simulink model "H8_6gdl_hil"  (R2022b)
settings: Solver=VariableStepAuto  StartTime=0.0  StopTime=10.0  RelTol=1e-3
InitFcn:
  | load("ems.mat");
  | load("hems.mat");
  | load('fuerzasY_LIM.mat')
  | load('matrices_linealizacion_6gdl.mat')
  | m = 200;
  | g = 9.81;
  | 
  | x_lev12 = 0.50086;
  | x_lev34 = 0.48414;
  | x_guid12 = 0.50503;
  | x_guid34 = 0.48831;
  | x_lim = 0.00778;
  | 
  | y_lev13 = 0.23523;
  | y_lev24 = 0.23827;
  | y_guid13 = 0.2372;
  | y_guid24 = 0.2402;
  | y_lim = 0.00154;
  | y_brk = 0.21552;
  | 
  | z_lev = 0.07138;
  | z_guid = 0.04113;
  | z_lim = 0.09146;
  | z_brk = 0.03941;
  | 
  | kp_lev = 50;
  | ki_lev = 400;
  | kp_guid = 6;
  | ki_guid = 46.5;
  | 
  | Imax_lev = 50;
  | Imin_lev = -50;
  | Imax_guid = 50;
  | Imin_guid = 0;
  | 
  | cg_nom=0.61448;
  | lev_nom=0.01965;
  | cg_suelo=0.61733;
  | cg_techo=0.60483;
  | 
  | I = [43.082 0 0; 0 26.887 -0; 0 0 29.297];
undefined symbols (not defined in the file or in its folder): current, ems, FuerzaRail_Y, hems, magnitude, Y
settings Model: Creator=aceao  LastModifiedBy=aceao

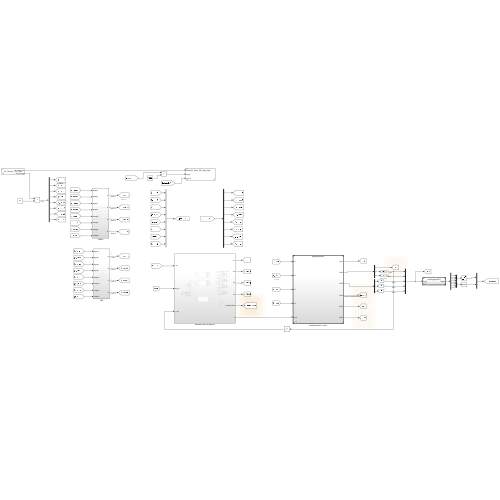
[thumbnail: Simulink's stored preview of the top-level diagram]
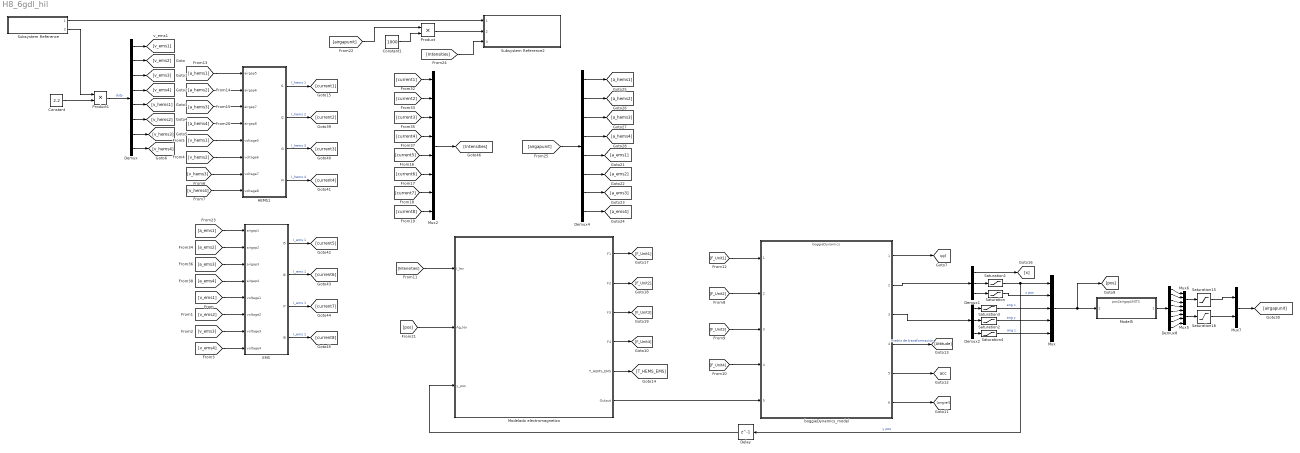
== system H8_6gdl_hil ==
  Constant : Constant  Value=2.2
  Constant1 : Constant  Value=1000
  Delay : Delay  DelayLength=1  InitialCondition=0.001
  Demux : Demux  Outputs=8
  Demux1 : Demux  Outputs=3
  Demux2 : Demux  Outputs=3
  Demux4 : Demux  Outputs=8
  Demux8 : Demux  Outputs=8
  EMS : Subsystem
  HEMS1 : Subsystem
  Model5 : ModelReference  ModelNameDialog=pos2airgapUNITS.slx  SimulationMode=Normal  ModelReferenceVersion=1.5
  Modelado electromagnetico : Subsystem
  Mux : Mux  Inputs=5
  Mux2 : Mux  Inputs=8
  Mux5 : Mux
  Mux6 : Mux
  Mux7 : Mux  Inputs=2
  Product : Product
  Product1 : Product
  Saturation : Saturate  UpperLimit=cg_suelo  LowerLimit=cg_techo
  Saturation1 : Saturate  UpperLimit=0.012  LowerLimit=-0.012
  Saturation15 : Saturate  UpperLimit=0.0225  LowerLimit=0.01
  Saturation16 : Saturate  UpperLimit=0.024  LowerLimit=0
  Saturation2 : Saturate  UpperLimit=0.01268  LowerLimit=-0.01268
  Saturation3 : Saturate  UpperLimit=0.0476  LowerLimit=-0.0476
  Saturation4 : Saturate  UpperLimit=0.024  LowerLimit=-0.024
  Subsystem Reference : Subsystem  ReferencedSubsystem=HIL_Receive_TCP_Data  mi_ip=0  mi_port=0  f=0
  Subsystem Reference2 : Subsystem  ReferencedSubsystem=HIL_Send_TCP_Data_6gdl  mi_ip=mi_ip  mi_port=mi_port  f=0
  boggieDynamics_model : ModelReference  ModelNameDialog=boggieDynamics.mdl  SimulationMode=Normal  ModelReferenceVersion=1.43
  tag scope: acc=global, vel=global
  wires:
  Mux2/1 -> [Intensities]
  [current5] -> Mux2/5
  [a_hems4] -> HEMS1/4(airgap8)
  [current2] -> Mux2/2
  HEMS1/1(I1) -> [current1]  "I_hems 1"
  [current6] -> Mux2/6
  [current7] -> Mux2/7
  [a_hems1] -> HEMS1/1(airgap5)
  HEMS1/4(I4) -> [current4]  "I_hems 4"
  [current1] -> Mux2/1
  HEMS1/2(I2) -> [current2]  "I_hems 2"
  [a_hems2] -> HEMS1/2(airgap6)
  [a_hems3] -> HEMS1/3(airgap7)
  [current3] -> Mux2/3
  HEMS1/3(I3) -> [current3]  "I_hems 3"
  [current8] -> Mux2/8
  [current4] -> Mux2/4
  Subsystem Reference/1 -> Subsystem Reference2/1
  [a_ems3] -> EMS/3(airgap3)
  [a_ems1] -> EMS/1(airgap1)
  [a_ems4] -> EMS/4(airgap4)
  [a_ems2] -> EMS/2(airgap2)
  EMS/4(I8) -> [current8]  "I_ems 1"
  EMS/3(I7) -> [current7]  "I_ems 1"
  EMS/1(I5) -> [current5]  "I_ems 1"
  EMS/2(I6) -> [current6]  "I_ems 1"
  Product1/1 -> Demux/1  "duty"
  Subsystem Reference/2 -> Product1/1
  Constant/1 -> Product1/2
  [v_ems1] -> EMS/5(voltage1)
  [v_ems2] -> EMS/6(voltage2)
  [v_ems3] -> EMS/7(voltage3)
  [v_ems4] -> EMS/8(voltage4)
  Demux/1 -> [v_ems1]
  Demux/2 -> [v_ems2]
  Demux/3 -> [v_ems3]
  Demux/4 -> [v_ems4]
  Demux/5 -> [v_hems1]
  Demux/6 -> [v_hems2]
  [v_hems1] -> HEMS1/5(voltage5)
  [v_hems2] -> HEMS1/6(voltage6)
  [v_hems3] -> HEMS1/7(voltage7)
  Demux/7 -> [v_hems3]
  [v_hems4] -> HEMS1/8(voltage8)
  Demux/8 -> [v_hems4]
  Modelado electromagnetico/3(F3) -> [F_Unit3]
  boggieDynamics_model/6 -> [angvel]
  Demux1/2 -> Saturation1/1
  Delay/1 -> Modelado electromagnetico/3(y_pos)
  Modelado electromagnetico/6(Output) -> boggieDynamics_model/5
  Demux2/1 -> Saturation3/1
  Saturation2/1 -> Mux/4  "ang y"
  [Intensities] -> Modelado electromagnetico/1(I_lev)
  Saturation4/1 -> Mux/5  "ang z"
  Saturation1/1 -> Delay/1, Mux/1  "y pos"
  boggieDynamics_model/2 -> Demux1/1
  Demux2/2 -> Saturation2/1
  Modelado electromagnetico/1(F1) -> [F_Unit1]
  Saturation3/1 -> Mux/3  "ang x"
  Modelado electromagnetico/5(T_HEMS_EMS) -> [T_HEMS_EMS]
  boggieDynamics_model/5 -> [acc]
  [F_Unit2] -> boggieDynamics_model/2
  Saturation/1 -> Mux/2  "z pos"
  Mux/1 -> Model5/1, [pos]
  boggieDynamics_model/4 -> [Attitude]  "matriz de transformacion"
  [F_Unit1] -> boggieDynamics_model/1
  Demux1/3 -> Saturation/1
  [F_Unit3] -> boggieDynamics_model/3
  Demux2/3 -> Saturation4/1
  [pos] -> Modelado electromagnetico/2(Ag_lev)
  Modelado electromagnetico/4(F4) -> [F_Unit4]
  Modelado electromagnetico/2(F2) -> [F_Unit2]
  [F_Unit4] -> boggieDynamics_model/4
  Demux1/1 -> [x]
  boggieDynamics_model/3 -> Demux2/1
  boggieDynamics_model/1 -> [vel]
  [Intensities] -> Subsystem Reference2/3
  Demux4/8 -> [a_ems4]
  Demux4/4 -> [a_hems4]
  Demux4/5 -> [a_ems1]
  [airgapunit] -> Demux4/1
  Demux4/6 -> [a_ems2]
  Demux4/3 -> [a_hems3]
  Demux4/2 -> [a_hems2]
  Demux4/1 -> [a_hems1]
  Demux4/7 -> [a_ems3]
  Mux7/1 -> [airgapunit]
  Demux8/6 -> Mux5/2
  Demux8/8 -> Mux5/4
  Demux8/1 -> Mux6/1
  Demux8/4 -> Mux6/4
  Model5/1 -> Demux8/1
  Demux8/7 -> Mux5/3
  Saturation15/1 -> Mux7/1
  Demux8/3 -> Mux6/3
  Mux5/1 -> Saturation16/1
  Mux6/1 -> Saturation15/1
  Demux8/5 -> Mux5/1
  Demux8/2 -> Mux6/2
  Saturation16/1 -> Mux7/2
  Constant1/1 -> Product/2
  [airgapunit] -> Product/1
  Product/1 -> Subsystem Reference2/2

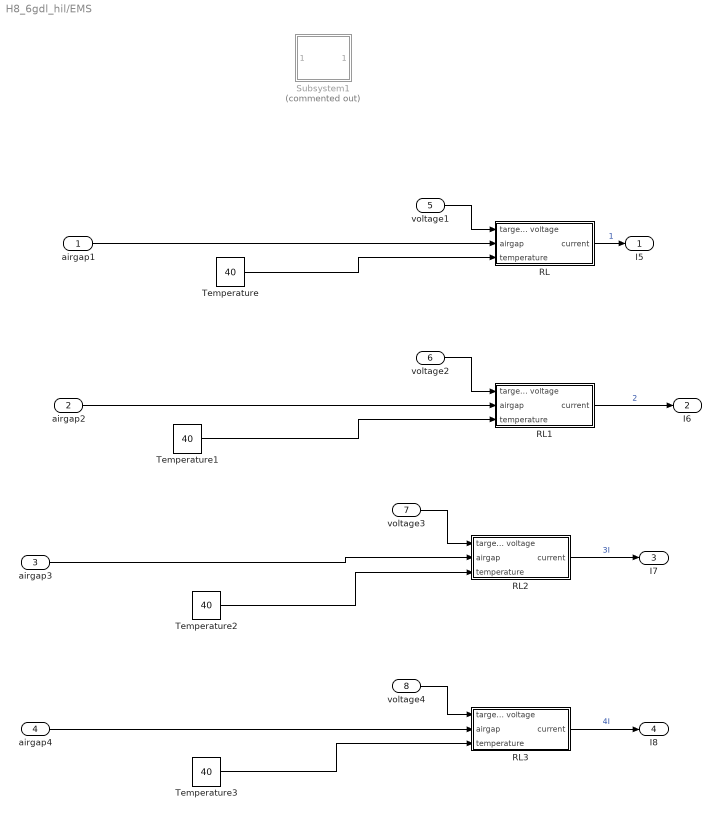
== system H8_6gdl_hil/EMS ==
  airgap1 : Inport
  airgap2 : Inport  Port=2
  airgap3 : Inport  Port=3
  airgap4 : Inport  Port=4
  voltage1 : Inport  Port=5
  voltage2 : Inport  Port=6
  voltage3 : Inport  Port=7
  voltage4 : Inport  Port=8
  RL : Subsystem
  RL1 : Subsystem
  RL2 : Subsystem
  RL3 : Subsystem
  Subsystem1 : Subsystem  Commented=on
  Temperature{,1..3} (4 alike) : Constant  Value=40
  I5 : Outport
  I6 : Outport  Port=2
  I7 : Outport  Port=3
  I8 : Outport  Port=4
  wires:
  Temperature/1 -> RL/3(temperature)
  airgap1/1 -> RL/2(airgap)
  Temperature3/1 -> RL3/3(temperature)
  RL/1(current) -> I5/1  "1"
  Temperature1/1 -> RL1/3(temperature)
  Temperature2/1 -> RL2/3(temperature)
  RL3/1(current) -> I8/1  "4I"
  airgap2/1 -> RL1/2(airgap)
  RL1/1(current) -> I6/1  "2"
  RL2/1(current) -> I7/1  "3I"
  airgap3/1 -> RL2/2(airgap)
  airgap4/1 -> RL3/2(airgap)
  voltage2/1 -> RL1/1(target voltage)
  voltage3/1 -> RL2/1(target voltage)
  voltage1/1 -> RL/1(target voltage)
  voltage4/1 -> RL3/1(target voltage)

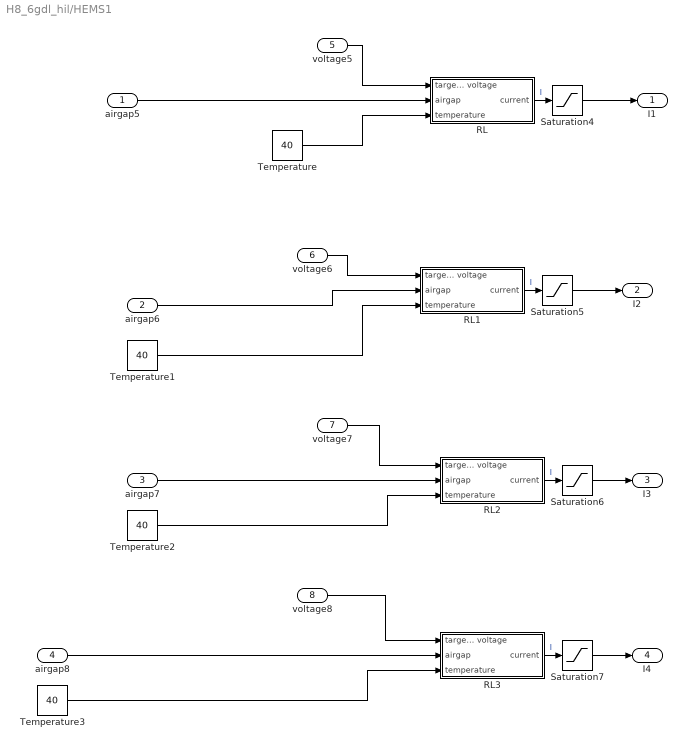
== system H8_6gdl_hil/HEMS1 ==
  airgap5 : Inport
  airgap6 : Inport  Port=2
  airgap7 : Inport  Port=3
  airgap8 : Inport  Port=4
  voltage5 : Inport  Port=5
  voltage6 : Inport  Port=6
  voltage7 : Inport  Port=7
  voltage8 : Inport  Port=8
  RL : Subsystem
  RL1 : Subsystem
  RL2 : Subsystem
  RL3 : Subsystem
  Saturation{4..7} (4 alike) : Saturate  UpperLimit=50  LowerLimit=-50
  Temperature{,1..3} (4 alike) : Constant  Value=40
  I1 : Outport
  I2 : Outport  Port=2
  I3 : Outport  Port=3
  I4 : Outport  Port=4
  wires:
  Temperature/1 -> RL/3(temperature)
  airgap5/1 -> RL/2(airgap)
  Temperature3/1 -> RL3/3(temperature)
  RL/1(current) -> Saturation4/1  "I"
  Temperature1/1 -> RL1/3(temperature)
  Temperature2/1 -> RL2/3(temperature)
  RL3/1(current) -> Saturation7/1  "I"
  airgap6/1 -> RL1/2(airgap)
  RL1/1(current) -> Saturation5/1  "I"
  RL2/1(current) -> Saturation6/1  "I"
  airgap7/1 -> RL2/2(airgap)
  airgap8/1 -> RL3/2(airgap)
  Saturation4/1 -> I1/1
  Saturation5/1 -> I2/1
  Saturation7/1 -> I4/1
  Saturation6/1 -> I3/1
  voltage5/1 -> RL/1(target voltage)
  voltage6/1 -> RL1/1(target voltage)
  voltage7/1 -> RL2/1(target voltage)
  voltage8/1 -> RL3/1(target voltage)

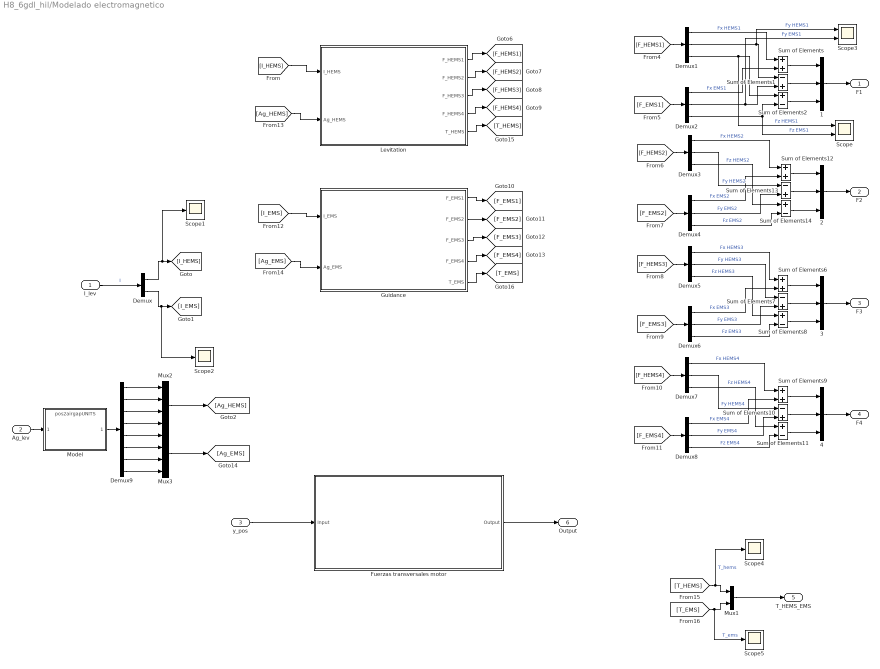
== system H8_6gdl_hil/Modelado electromagnetico ==
  I_lev : Inport
  Ag_lev : Inport  Port=2
  y_pos : Inport  Port=3
  {1..4} (4 alike) : Mux  Inputs=3
  Demux : Demux  Outputs=2
  Demux{1..8} (8 alike) : Demux  Outputs=3
  Demux9 : Demux  Outputs=8
  Fuerzas transversales motor : Subsystem
  Guidance : Subsystem
  Levitation : Subsystem
  Model : ModelReference  ModelNameDialog=pos2airgapUNITS.slx  SimulationMode=Normal  ModelReferenceVersion=1.5
  Mux1 : Mux  Inputs=2
  Mux2 : Mux
  Mux3 : Mux
  Scope : Scope  NumInputPorts=2
  Scope{1..2,4..5} (4 alike) : Scope
  Scope3 : Scope  NumInputPorts=2
  Sum of Elements{,6,9,12} (4 alike) : Sum
  Sum of Elements{1,7,10,13} (4 alike) : Sum  Inputs=-+
  Sum of Elements{2,8,11,14} (4 alike) : Sum  Inputs=+-
  F1 : Outport
  F2 : Outport  Port=2
  F3 : Outport  Port=3
  F4 : Outport  Port=4
  T_HEMS_EMS : Outport  Port=5
  Output : Outport  Port=6
  wires:
  I_lev/1 -> Demux/1  "I"
  Demux/1 -> Scope1/1, [I_HEMS]
  Demux/2 -> Scope2/1, [I_EMS]
  [I_HEMS] -> Levitation/1(I_HEMS)
  Levitation/1(F_HEMS1) -> [F_HEMS1]
  Levitation/2(F_HEMS2) -> [F_HEMS2]
  Levitation/3(F_HEMS3) -> [F_HEMS3]
  Levitation/4(F_HEMS4) -> [F_HEMS4]
  Sum of Elements/1 -> 1/1
  1/1 -> F1/1
  Sum of Elements1/1 -> 1/2
  Sum of Elements2/1 -> 1/3
  2/1 -> F2/1
  [F_HEMS1] -> Demux1/1
  Demux1/1 -> Sum of Elements/1  "Fx HEMS1"
  Demux1/2 -> Scope3/1, Sum of Elements1/1  "Fy HEMS1"
  Demux1/3 -> Scope/1, Sum of Elements2/1  "Fz HEMS1"
  3/1 -> F3/1
  Sum of Elements8/1 -> 3/3
  Sum of Elements6/1 -> 3/1
  Sum of Elements7/1 -> 3/2
  4/1 -> F4/1
  Sum of Elements11/1 -> 4/3
  Sum of Elements9/1 -> 4/1
  Sum of Elements10/1 -> 4/2
  Guidance/2(F_EMS2) -> [F_EMS2]
  Guidance/3(F_EMS3) -> [F_EMS3]
  Guidance/4(F_EMS4) -> [F_EMS4]
  Guidance/1(F_EMS1) -> [F_EMS1]
  Demux2/1 -> Sum of Elements/2  "Fx EMS1"
  [F_EMS1] -> Demux2/1
  Demux2/2 -> Scope3/2, Sum of Elements1/2  "Fy EMS1"
  Demux2/3 -> Sum of Elements2/2, Scope/2  "Fz EMS1"
  [F_EMS2] -> Demux4/1
  Demux4/1 -> Sum of Elements12/2  "Fx EMS2"
  Demux4/2 -> Sum of Elements13/2  "Fy EMS2"
  Sum of Elements14/1 -> 2/3
  Demux3/1 -> Sum of Elements12/1  "Fx HEMS2"
  [F_HEMS2] -> Demux3/1
  Demux3/2 -> Sum of Elements13/1  "Fy HEMS2"
  Demux3/3 -> Sum of Elements14/1  "Fz HEMS2"
  Sum of Elements13/1 -> 2/2
  Sum of Elements12/1 -> 2/1
  Demux4/3 -> Sum of Elements14/2  "Fz EMS2"
  Demux5/3 -> Sum of Elements8/1  "Fz HEMS3"
  Demux5/2 -> Sum of Elements7/1  "Fy HEMS3"
  [F_HEMS3] -> Demux5/1
  Demux6/3 -> Sum of Elements8/2  "Fz EMS3"
  [F_EMS3] -> Demux6/1
  Demux6/1 -> Sum of Elements6/2  "Fx EMS3"
  Demux5/1 -> Sum of Elements6/1  "Fx HEMS3"
  Demux6/2 -> Sum of Elements7/2  "Fy EMS3"
  Demux7/3 -> Sum of Elements11/1  "Fz HEMS4"
  Demux8/3 -> Sum of Elements11/2  "Fz EMS4"
  Demux8/2 -> Sum of Elements10/2  "Fy EMS4"
  Demux7/2 -> Sum of Elements10/1  "Fy HEMS4"
  Demux7/1 -> Sum of Elements9/1  "Fx HEMS4"
  Demux8/1 -> Sum of Elements9/2  "Fx EMS4"
  [F_HEMS4] -> Demux7/1
  [F_EMS4] -> Demux8/1
  [I_EMS] -> Guidance/1(I_EMS)
  Ag_lev/1 -> Model/1
  [Ag_HEMS] -> Levitation/2(Ag_HEMS)
  [Ag_EMS] -> Guidance/2(Ag_EMS)
  Levitation/5(T_HEMS) -> [T_HEMS]
  Guidance/5(T_EMS) -> [T_EMS]
  Mux1/1 -> T_HEMS_EMS/1
  [T_HEMS] -> Scope4/1, Mux1/1  "T_hems"
  [T_EMS] -> Scope5/1, Mux1/2  "T_ems"
  Model/1 -> Demux9/1
  Demux9/1 -> Mux2/1
  Demux9/2 -> Mux2/2
  Demux9/3 -> Mux2/3
  Demux9/4 -> Mux2/4
  Mux2/1 -> [Ag_HEMS]
  Demux9/5 -> Mux3/1
  Demux9/7 -> Mux3/3
  Mux3/1 -> [Ag_EMS]
  Demux9/6 -> Mux3/2
  Demux9/8 -> Mux3/4
  y_pos/1 -> Fuerzas transversales motor/1(Input)
  Fuerzas transversales motor/1(Output) -> Output/1

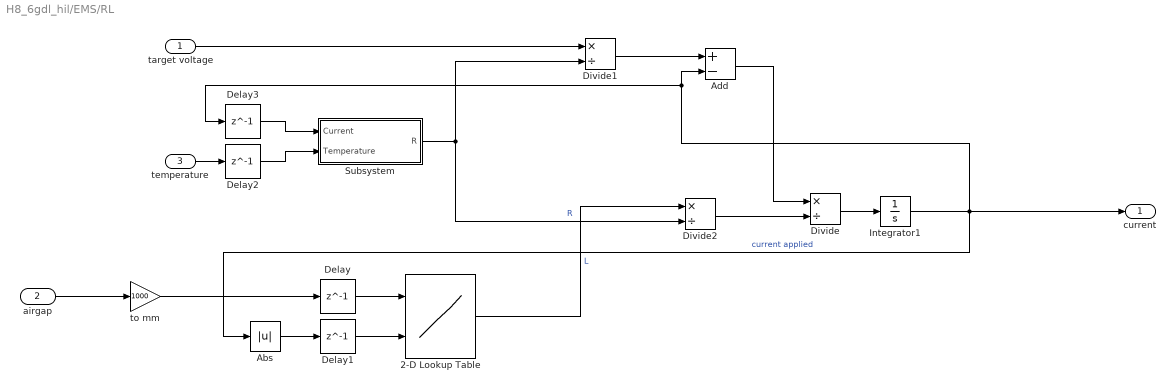
== system H8_6gdl_hil/EMS/RL ==
  target voltage : Inport
  airgap : Inport  Port=2
  temperature : Inport  Port=3
  2-D Lookup Table : Lookup_n-D  BreakpointsForDimension1=ems.Airgap  BreakpointsForDimension2=ems.Flux_Current(2:55)  Table=ems.Inductance  InternalRulePriority=Speed  RndMeth=Simplest
      settings: InputPortMap=u0,u1
  Abs : Abs  SaturateOnIntegerOverflow=off
  Add : Sum  Inputs=+-
  Delay{,1..3} (4 alike) : Delay  DelayLength=1
  Divide : Product  Inputs=*/
  Divide1 : Product  Inputs=*/
  Divide2 : Product  Inputs=*/
  Integrator1 : Integrator
  Subsystem : Subsystem
  to mm : Gain  Gain=1000
  current : Outport
  wires:
  airgap/1 -> to mm/1
  Divide/1 -> Integrator1/1
  Add/1 -> Divide/1
  Integrator1/1 -> Abs/1, current/1, Delay3/1, Add/2  "current applied"
  2-D Lookup Table/1 -> Divide2/1  "L"
  target voltage/1 -> Divide1/1
  temperature/1 -> Delay2/1
  Divide1/1 -> Add/1
  Subsystem/1(R) -> Divide2/2, Divide1/2  "R"
  Delay3/1 -> Subsystem/1(Current)
  Delay2/1 -> Subsystem/2(Temperature)
  Divide2/1 -> Divide/2
  Delay1/1 -> 2-D Lookup Table/2
  Delay/1 -> 2-D Lookup Table/1
  Abs/1 -> Delay1/1
  to mm/1 -> Delay/1

== system H8_6gdl_hil/EMS/RL1 ==
  target voltage : Inport
  airgap : Inport  Port=2
  temperature : Inport  Port=3
  2-D Lookup Table : Lookup_n-D  BreakpointsForDimension1=ems.Airgap  BreakpointsForDimension2=ems.Flux_Current(2:55)  Table=ems.Inductance  InternalRulePriority=Speed  RndMeth=Simplest
      settings: InputPortMap=u0,u1
  Abs : Abs  SaturateOnIntegerOverflow=off
  Add : Sum  Inputs=+-
  Delay{,1..3} (4 alike) : Delay  DelayLength=1
  Divide : Product  Inputs=*/
  Divide1 : Product  Inputs=*/
  Divide2 : Product  Inputs=*/
  Integrator1 : Integrator
  Subsystem : Subsystem
  to mm : Gain  Gain=1000
  current : Outport
  wires:
  airgap/1 -> to mm/1
  Divide/1 -> Integrator1/1
  Add/1 -> Divide/1
  Integrator1/1 -> Abs/1, current/1, Delay3/1, Add/2  "current applied"
  2-D Lookup Table/1 -> Divide2/1  "L"
  target voltage/1 -> Divide1/1
  temperature/1 -> Delay2/1
  Divide1/1 -> Add/1
  Subsystem/1(R) -> Divide2/2, Divide1/2  "R"
  Delay3/1 -> Subsystem/1(Current)
  Delay2/1 -> Subsystem/2(Temperature)
  Divide2/1 -> Divide/2
  Delay1/1 -> 2-D Lookup Table/2
  Delay/1 -> 2-D Lookup Table/1
  Abs/1 -> Delay1/1
  to mm/1 -> Delay/1

== system H8_6gdl_hil/EMS/RL2 ==
  target voltage : Inport
  airgap : Inport  Port=2
  temperature : Inport  Port=3
  2-D Lookup Table : Lookup_n-D  BreakpointsForDimension1=ems.Airgap  BreakpointsForDimension2=ems.Flux_Current(2:55)  Table=ems.Inductance  InternalRulePriority=Speed  RndMeth=Simplest
      settings: InputPortMap=u0,u1
  Abs : Abs  SaturateOnIntegerOverflow=off
  Add : Sum  Inputs=+-
  Delay{,1..3} (4 alike) : Delay  DelayLength=1
  Divide : Product  Inputs=*/
  Divide1 : Product  Inputs=*/
  Divide2 : Product  Inputs=*/
  Integrator1 : Integrator
  Subsystem : Subsystem
  to mm : Gain  Gain=1000
  current : Outport
  wires:
  airgap/1 -> to mm/1
  Divide/1 -> Integrator1/1
  Add/1 -> Divide/1
  Integrator1/1 -> Abs/1, current/1, Delay3/1, Add/2  "current applied"
  2-D Lookup Table/1 -> Divide2/1  "L"
  target voltage/1 -> Divide1/1
  temperature/1 -> Delay2/1
  Divide1/1 -> Add/1
  Subsystem/1(R) -> Divide2/2, Divide1/2  "R"
  Delay3/1 -> Subsystem/1(Current)
  Delay2/1 -> Subsystem/2(Temperature)
  Divide2/1 -> Divide/2
  Delay1/1 -> 2-D Lookup Table/2
  Delay/1 -> 2-D Lookup Table/1
  Abs/1 -> Delay1/1
  to mm/1 -> Delay/1

== system H8_6gdl_hil/EMS/RL3 ==
  target voltage : Inport
  airgap : Inport  Port=2
  temperature : Inport  Port=3
  2-D Lookup Table : Lookup_n-D  BreakpointsForDimension1=ems.Airgap  BreakpointsForDimension2=ems.Flux_Current(2:55)  Table=ems.Inductance  InternalRulePriority=Speed  RndMeth=Simplest
      settings: InputPortMap=u0,u1
  Abs : Abs  SaturateOnIntegerOverflow=off
  Add : Sum  Inputs=+-
  Delay{,1..3} (4 alike) : Delay  DelayLength=1
  Divide : Product  Inputs=*/
  Divide1 : Product  Inputs=*/
  Divide2 : Product  Inputs=*/
  Integrator1 : Integrator
  Subsystem : Subsystem
  to mm : Gain  Gain=1000
  current : Outport
  wires:
  airgap/1 -> to mm/1
  Divide/1 -> Integrator1/1
  Add/1 -> Divide/1
  Integrator1/1 -> Abs/1, current/1, Delay3/1, Add/2  "current applied"
  2-D Lookup Table/1 -> Divide2/1  "L"
  target voltage/1 -> Divide1/1
  temperature/1 -> Delay2/1
  Divide1/1 -> Add/1
  Subsystem/1(R) -> Divide2/2, Divide1/2  "R"
  Delay3/1 -> Subsystem/1(Current)
  Delay2/1 -> Subsystem/2(Temperature)
  Divide2/1 -> Divide/2
  Delay1/1 -> 2-D Lookup Table/2
  Delay/1 -> 2-D Lookup Table/1
  Abs/1 -> Delay1/1
  to mm/1 -> Delay/1

== system H8_6gdl_hil/EMS/Subsystem1 ==
  current5 : Inport
  Constant : Constant  Value=0
  Constant2 : Constant  Value=50
  Switch : Switch  Criteria=u2 > Threshold  SaturateOnIntegerOverflow=off  InputSameDT=off
  Switch1 : Switch  Criteria=u2 > Threshold  Threshold=50  SaturateOnIntegerOverflow=off  InputSameDT=off
  Out1 : Outport
  wires:
  current5/1 -> Switch/1, Switch/2
  Switch1/1 -> Out1/1
  Switch/1 -> Switch1/3, Switch1/2
  Constant/1 -> Switch/3
  Constant2/1 -> Switch1/1

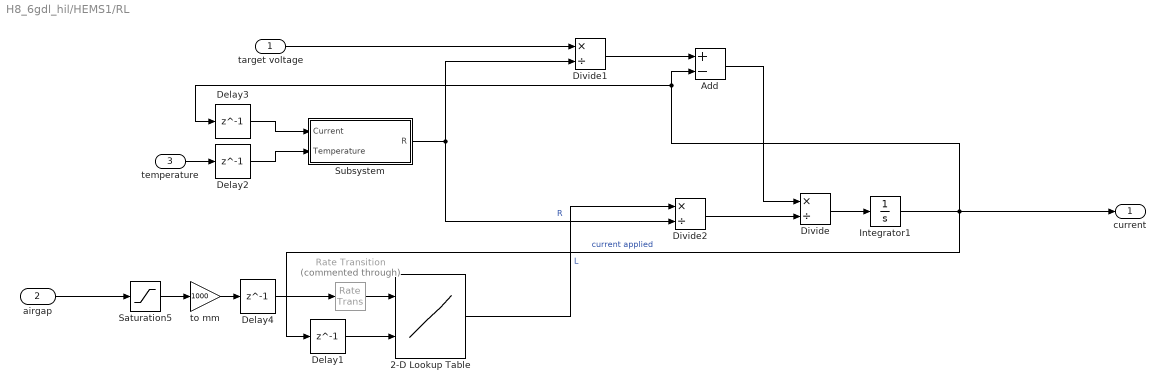
== system H8_6gdl_hil/HEMS1/RL ==
  target voltage : Inport
  airgap : Inport  Port=2
  temperature : Inport  Port=3
  2-D Lookup Table : Lookup_n-D  BreakpointsForDimension1=hems.Airgap  BreakpointsForDimension2=hems.Current(2:110)  Table=hems.Inductance  InternalRulePriority=Speed  RndMeth=Simplest
      settings: InputPortMap=u0,u1
  Add : Sum  Inputs=+-
  Delay{1..4} (4 alike) : Delay  DelayLength=1
  Divide : Product  Inputs=*/
  Divide1 : Product  Inputs=*/
  Divide2 : Product  Inputs=*/
  Integrator1 : Integrator
  Rate Transition : RateTransition  Commented=through
  Saturation5 : Saturate  UpperLimit=0.0225  LowerLimit=0.01
  Subsystem : Subsystem
  to mm : Gain  Gain=1000
  current : Outport
  wires:
  airgap/1 -> Saturation5/1
  Divide/1 -> Integrator1/1
  Add/1 -> Divide/1
  Integrator1/1 -> Delay1/1, current/1, Delay3/1, Add/2  "current applied"
  2-D Lookup Table/1 -> Divide2/1  "L"
  temperature/1 -> Delay2/1
  Divide1/1 -> Add/1
  Subsystem/1(R) -> Divide2/2, Divide1/2  "R"
  Delay3/1 -> Subsystem/1(Current)
  Delay2/1 -> Subsystem/2(Temperature)
  Divide2/1 -> Divide/2
  Delay1/1 -> 2-D Lookup Table/2
  Rate Transition/1 -> 2-D Lookup Table/1
  Saturation5/1 -> to mm/1
  to mm/1 -> Delay4/1
  Delay4/1 -> Rate Transition/1
  target voltage/1 -> Divide1/1

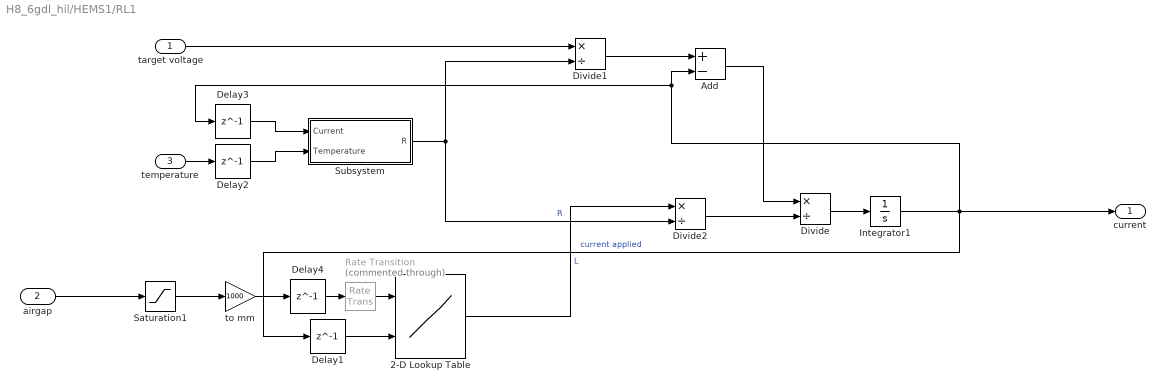
== system H8_6gdl_hil/HEMS1/RL1 ==
  target voltage : Inport
  airgap : Inport  Port=2
  temperature : Inport  Port=3
  2-D Lookup Table : Lookup_n-D  BreakpointsForDimension1=hems.Airgap  BreakpointsForDimension2=hems.Current(2:110)  Table=hems.Inductance  InternalRulePriority=Speed  RndMeth=Simplest
      settings: InputPortMap=u0,u1
  Add : Sum  Inputs=+-
  Delay{1..4} (4 alike) : Delay  DelayLength=1
  Divide : Product  Inputs=*/
  Divide1 : Product  Inputs=*/
  Divide2 : Product  Inputs=*/
  Integrator1 : Integrator
  Rate Transition : RateTransition  Commented=through
  Saturation1 : Saturate  UpperLimit=0.0225  LowerLimit=0.01
  Subsystem : Subsystem
  to mm : Gain  Gain=1000
  current : Outport
  wires:
  airgap/1 -> Saturation1/1
  Divide/1 -> Integrator1/1
  Add/1 -> Divide/1
  Integrator1/1 -> Delay1/1, current/1, Delay3/1, Add/2  "current applied"
  2-D Lookup Table/1 -> Divide2/1  "L"
  target voltage/1 -> Divide1/1
  temperature/1 -> Delay2/1
  Divide1/1 -> Add/1
  Subsystem/1(R) -> Divide2/2, Divide1/2  "R"
  Delay3/1 -> Subsystem/1(Current)
  Delay2/1 -> Subsystem/2(Temperature)
  Divide2/1 -> Divide/2
  Delay1/1 -> 2-D Lookup Table/2
  Rate Transition/1 -> 2-D Lookup Table/1
  Saturation1/1 -> to mm/1
  to mm/1 -> Delay4/1
  Delay4/1 -> Rate Transition/1

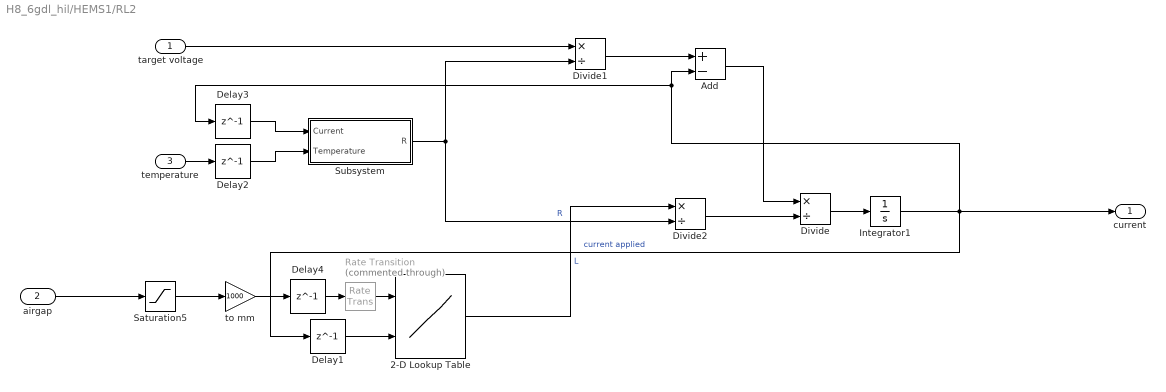
== system H8_6gdl_hil/HEMS1/RL2 ==
  target voltage : Inport
  airgap : Inport  Port=2
  temperature : Inport  Port=3
  2-D Lookup Table : Lookup_n-D  BreakpointsForDimension1=hems.Airgap  BreakpointsForDimension2=hems.Current(2:110)  Table=hems.Inductance  InternalRulePriority=Speed  RndMeth=Simplest
      settings: InputPortMap=u0,u1
  Add : Sum  Inputs=+-
  Delay{1..4} (4 alike) : Delay  DelayLength=1
  Divide : Product  Inputs=*/
  Divide1 : Product  Inputs=*/
  Divide2 : Product  Inputs=*/
  Integrator1 : Integrator
  Rate Transition : RateTransition  Commented=through
  Saturation5 : Saturate  UpperLimit=0.0225  LowerLimit=0.01
  Subsystem : Subsystem
  to mm : Gain  Gain=1000
  current : Outport
  wires:
  airgap/1 -> Saturation5/1
  Divide/1 -> Integrator1/1
  Add/1 -> Divide/1
  Integrator1/1 -> Delay1/1, current/1, Delay3/1, Add/2  "current applied"
  2-D Lookup Table/1 -> Divide2/1  "L"
  target voltage/1 -> Divide1/1
  temperature/1 -> Delay2/1
  Divide1/1 -> Add/1
  Subsystem/1(R) -> Divide2/2, Divide1/2  "R"
  Delay3/1 -> Subsystem/1(Current)
  Delay2/1 -> Subsystem/2(Temperature)
  Divide2/1 -> Divide/2
  Delay1/1 -> 2-D Lookup Table/2
  Rate Transition/1 -> 2-D Lookup Table/1
  Saturation5/1 -> to mm/1
  to mm/1 -> Delay4/1
  Delay4/1 -> Rate Transition/1

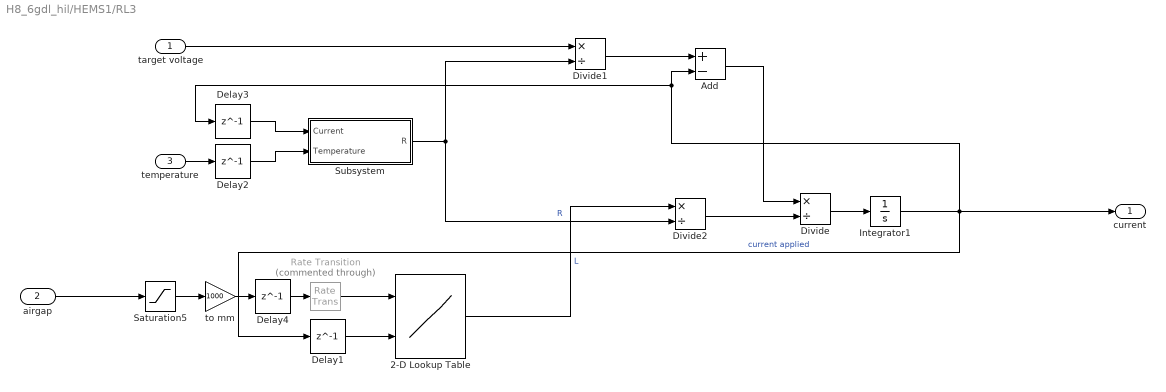
== system H8_6gdl_hil/HEMS1/RL3 ==
  target voltage : Inport
  airgap : Inport  Port=2
  temperature : Inport  Port=3
  2-D Lookup Table : Lookup_n-D  BreakpointsForDimension1=hems.Airgap  BreakpointsForDimension2=hems.Current(2:110)  Table=hems.Inductance  InternalRulePriority=Speed  RndMeth=Simplest
      settings: InputPortMap=u0,u1
  Add : Sum  Inputs=+-
  Delay{1..4} (4 alike) : Delay  DelayLength=1
  Divide : Product  Inputs=*/
  Divide1 : Product  Inputs=*/
  Divide2 : Product  Inputs=*/
  Integrator1 : Integrator
  Rate Transition : RateTransition  Commented=through
  Saturation5 : Saturate  UpperLimit=0.0225  LowerLimit=0.01
  Subsystem : Subsystem
  to mm : Gain  Gain=1000
  current : Outport
  wires:
  airgap/1 -> Saturation5/1
  Divide/1 -> Integrator1/1
  Add/1 -> Divide/1
  Integrator1/1 -> Delay1/1, current/1, Delay3/1, Add/2  "current applied"
  2-D Lookup Table/1 -> Divide2/1  "L"
  target voltage/1 -> Divide1/1
  temperature/1 -> Delay2/1
  Divide1/1 -> Add/1
  Subsystem/1(R) -> Divide2/2, Divide1/2  "R"
  Delay3/1 -> Subsystem/1(Current)
  Delay2/1 -> Subsystem/2(Temperature)
  Divide2/1 -> Divide/2
  Delay1/1 -> 2-D Lookup Table/2
  Rate Transition/1 -> 2-D Lookup Table/1
  Saturation5/1 -> to mm/1
  to mm/1 -> Delay4/1
  Delay4/1 -> Rate Transition/1

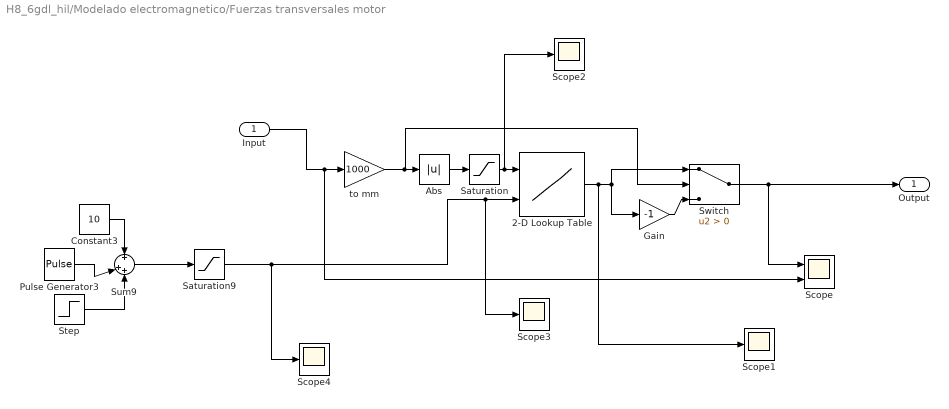
== system H8_6gdl_hil/Modelado electromagnetico/Fuerzas transversales motor ==
  Input : Inport
  2-D Lookup Table : Lookup_n-D  BreakpointsForDimension1=Y  BreakpointsForDimension2=current  Table=FuerzaRail_Y  InternalRulePriority=Speed  RndMeth=Simplest
      settings: InputPortMap=u0,u1
  Abs : Abs  SaturateOnIntegerOverflow=off
  Constant3 : Constant  Value=10
  Gain : Gain  Gain=-1
  Pulse Generator3 : DiscretePulseGenerator  PulseType=Time based  Amplitude=100  PulseWidth=95  PhaseDelay=1
  Saturation : Saturate  UpperLimit=6  LowerLimit=0
  Saturation9 : Saturate  UpperLimit=100  LowerLimit=0
  Scope : Scope  NumInputPorts=2
  Scope{1..4} (4 alike) : Scope
  Step : Step  Time=5  After=-100  SampleTime=0
  Sum9 : Sum  Inputs=+|++
  Switch : Switch  Criteria=u2 > Threshold  SaturateOnIntegerOverflow=off  InputSameDT=off
  to mm : Gain  Gain=1000
  Output : Outport
  wires:
  Input/1 -> to mm/1, Scope/2
  Gain/1 -> Switch/3
  Abs/1 -> Saturation/1
  to mm/1 -> Switch/2, Abs/1
  2-D Lookup Table/1 -> Scope1/1, Gain/1, Switch/1
  Saturation9/1 -> Scope4/1, Scope3/1, 2-D Lookup Table/2
  Switch/1 -> Output/1, Scope/1
  Saturation/1 -> Scope2/1, 2-D Lookup Table/1
  Sum9/1 -> Saturation9/1
  Pulse Generator3/1 -> Sum9/2
  Constant3/1 -> Sum9/1
  Step/1 -> Sum9/3

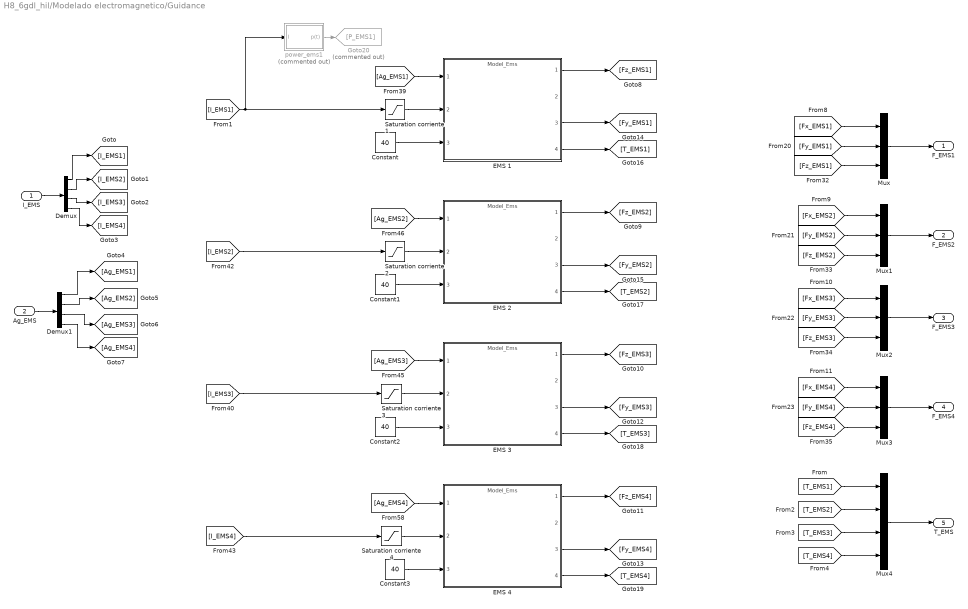
== system H8_6gdl_hil/Modelado electromagnetico/Guidance ==
  I_EMS : Inport
  Ag_EMS : Inport  Port=2
  Constant{,1..3} (4 alike) : Constant  Value=40
  Demux : Demux
  Demux1 : Demux
  EMS {1..4} (4 alike) : ModelReference  ModelNameDialog=Model_Ems.slx  SimulationMode=Normal  ModelReferenceVersion=1.23
  Goto20 : Goto  Commented=on  GotoTag=P_EMS1
  Mux{,1..3} (4 alike) : Mux  Inputs=3
  Mux4 : Mux
  Saturation corriente {1..4} (4 alike) : Saturate  UpperLimit=Imax_guid  LowerLimit=Imin_guid
  power_ems1 : Subsystem  Commented=on
  F_EMS1 : Outport
  F_EMS2 : Outport  Port=2
  F_EMS3 : Outport  Port=3
  F_EMS4 : Outport  Port=4
  T_EMS : Outport  Port=5
  wires:
  [Fz_EMS4] -> Mux3/3
  Demux1/4 -> [Ag_EMS4]
  [Fy_EMS1] -> Mux/2
  I_EMS/1 -> Demux/1
  Mux1/1 -> F_EMS2/1
  Demux/2 -> [I_EMS2]
  [Fy_EMS3] -> Mux2/2
  Mux3/1 -> F_EMS4/1
  [Fy_EMS4] -> Mux3/2
  [Fz_EMS1] -> Mux/3
  Mux/1 -> F_EMS1/1
  Mux2/1 -> F_EMS3/1
  [Fx_EMS3] -> Mux2/1
  Demux1/3 -> [Ag_EMS3]
  Ag_EMS/1 -> Demux1/1
  [Fz_EMS3] -> Mux2/3
  Demux/1 -> [I_EMS1]
  [Fz_EMS2] -> Mux1/3
  [Fx_EMS1] -> Mux/1
  Demux1/1 -> [Ag_EMS1]
  Demux/4 -> [I_EMS4]
  [Fx_EMS2] -> Mux1/1
  [Fy_EMS2] -> Mux1/2
  [Fx_EMS4] -> Mux3/1
  Demux/3 -> [I_EMS3]
  Demux1/2 -> [Ag_EMS2]
  EMS 1/3 -> [Fy_EMS1]
  [Ag_EMS4] -> EMS 4/1
  EMS 4/3 -> [Fy_EMS4]
  EMS 4/1 -> [Fz_EMS4]
  EMS 2/1 -> [Fz_EMS2]
  EMS 3/1 -> [Fz_EMS3]
  [Ag_EMS3] -> EMS 3/1
  Constant1/1 -> EMS 2/3
  Constant3/1 -> EMS 4/3
  Constant2/1 -> EMS 3/3
  Constant/1 -> EMS 1/3
  EMS 1/1 -> [Fz_EMS1]
  [Ag_EMS2] -> EMS 2/1
  EMS 3/3 -> [Fy_EMS3]
  EMS 2/3 -> [Fy_EMS2]
  [Ag_EMS1] -> EMS 1/1
  Mux4/1 -> T_EMS/1
  EMS 1/4 -> [T_EMS1]
  EMS 2/4 -> [T_EMS2]
  EMS 3/4 -> [T_EMS3]
  EMS 4/4 -> [T_EMS4]
  [T_EMS1] -> Mux4/1
  [T_EMS2] -> Mux4/2
  [T_EMS3] -> Mux4/3
  [T_EMS4] -> Mux4/4
  Saturation corriente 1/1 -> EMS 1/2
  Saturation corriente 2/1 -> EMS 2/2
  Saturation corriente 3/1 -> EMS 3/2
  Saturation corriente 4/1 -> EMS 4/2
  power_ems1/1(p(t)) -> Goto20/1
  [I_EMS4] -> Saturation corriente 4/1
  [I_EMS3] -> Saturation corriente 3/1
  [I_EMS2] -> Saturation corriente 2/1
  [I_EMS1] -> Saturation corriente 1/1, power_ems1/1(I)

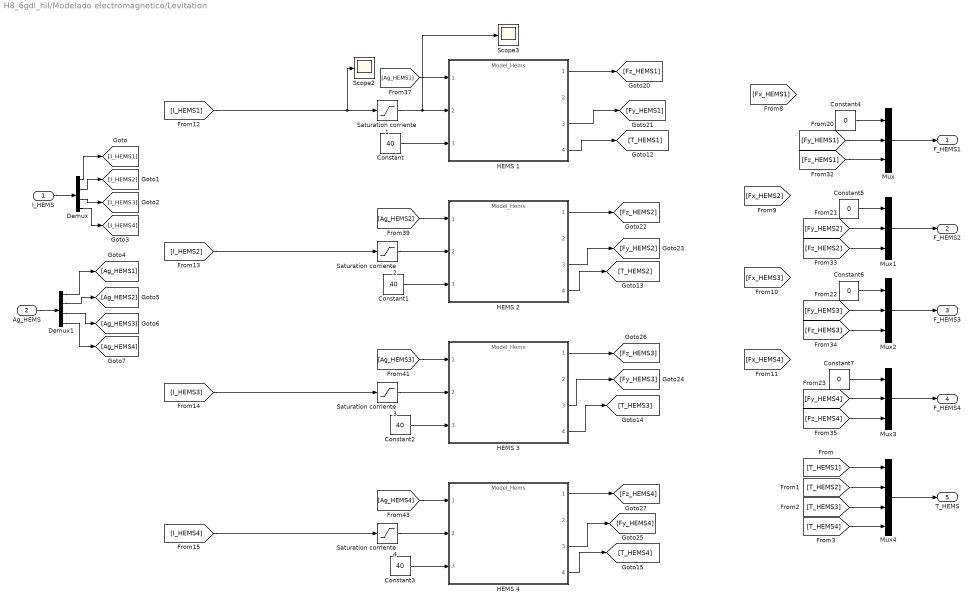
== system H8_6gdl_hil/Modelado electromagnetico/Levitation ==
  I_HEMS : Inport
  Ag_HEMS : Inport  Port=2
  Constant{,1..3} (4 alike) : Constant  Value=40
  Constant{4..7} (4 alike) : Constant  Value=0
  Demux : Demux
  Demux1 : Demux
  HEMS {1..4} (4 alike) : ModelReference  ModelNameDialog=Model_Hems.slx  SimulationMode=Normal  ModelReferenceVersion=1.26
  Mux{,1..3} (4 alike) : Mux  Inputs=3
  Mux4 : Mux
  Saturation corriente {1..4} (4 alike) : Saturate  UpperLimit=Imax_lev  LowerLimit=Imin_lev
  Scope2 : Scope
  Scope3 : Scope
  F_HEMS1 : Outport
  F_HEMS2 : Outport  Port=2
  F_HEMS3 : Outport  Port=3
  F_HEMS4 : Outport  Port=4
  T_HEMS : Outport  Port=5
  wires:
  I_HEMS/1 -> Demux/1
  Mux/1 -> F_HEMS1/1
  Mux1/1 -> F_HEMS2/1
  Mux2/1 -> F_HEMS3/1
  Mux3/1 -> F_HEMS4/1
  Demux/1 -> [I_HEMS1]
  Demux/2 -> [I_HEMS2]
  Demux/3 -> [I_HEMS3]
  Demux/4 -> [I_HEMS4]
  Demux1/2 -> [Ag_HEMS2]
  Demux1/3 -> [Ag_HEMS3]
  Ag_HEMS/1 -> Demux1/1
  Demux1/4 -> [Ag_HEMS4]
  Demux1/1 -> [Ag_HEMS1]
  Constant4/1 -> Mux/1
  Constant5/1 -> Mux1/1
  Constant6/1 -> Mux2/1
  Constant7/1 -> Mux3/1
  [Fy_HEMS1] -> Mux/2
  [Fy_HEMS2] -> Mux1/2
  [Fy_HEMS3] -> Mux2/2
  [Fy_HEMS4] -> Mux3/2
  [Fz_HEMS1] -> Mux/3
  [Fz_HEMS2] -> Mux1/3
  [Fz_HEMS3] -> Mux2/3
  [Fz_HEMS4] -> Mux3/3
  [Ag_HEMS1] -> HEMS 1/1
  HEMS 1/1 -> [Fz_HEMS1]
  HEMS 1/3 -> [Fy_HEMS1]
  HEMS 2/3 -> [Fy_HEMS2]
  HEMS 2/1 -> [Fz_HEMS2]
  [Ag_HEMS2] -> HEMS 2/1
  HEMS 3/3 -> [Fy_HEMS3]
  HEMS 3/1 -> [Fz_HEMS3]
  [Ag_HEMS3] -> HEMS 3/1
  HEMS 4/3 -> [Fy_HEMS4]
  HEMS 4/1 -> [Fz_HEMS4]
  [Ag_HEMS4] -> HEMS 4/1
  Constant1/1 -> HEMS 2/3
  Constant2/1 -> HEMS 3/3
  Constant3/1 -> HEMS 4/3
  HEMS 1/4 -> [T_HEMS1]
  Constant/1 -> HEMS 1/3
  HEMS 2/4 -> [T_HEMS2]
  HEMS 3/4 -> [T_HEMS3]
  HEMS 4/4 -> [T_HEMS4]
  Mux4/1 -> T_HEMS/1
  [T_HEMS1] -> Mux4/1
  [T_HEMS4] -> Mux4/4
  [T_HEMS3] -> Mux4/3
  [T_HEMS2] -> Mux4/2
  Saturation corriente 1/1 -> Scope3/1, HEMS 1/2
  Saturation corriente 2/1 -> HEMS 2/2
  Saturation corriente 3/1 -> HEMS 3/2
  Saturation corriente 4/1 -> HEMS 4/2
  [I_HEMS4] -> Saturation corriente 4/1
  [I_HEMS2] -> Saturation corriente 2/1
  [I_HEMS1] -> Scope2/1, Saturation corriente 1/1
  [I_HEMS3] -> Saturation corriente 3/1

== system H8_6gdl_hil/EMS/RL/Subsystem ==
  Current : Inport
  Temperature : Inport  Port=2
  Resistance : Constant  Value=ems.Resistance
  R : Outport
  wires:
  Resistance/1 -> R/1

== system H8_6gdl_hil/EMS/RL1/Subsystem ==
  Current : Inport
  Temperature : Inport  Port=2
  Resistance : Constant  Value=ems.Resistance
  R : Outport
  wires:
  Resistance/1 -> R/1

== system H8_6gdl_hil/EMS/RL2/Subsystem ==
  Current : Inport
  Temperature : Inport  Port=2
  Resistance : Constant  Value=ems.Resistance
  R : Outport
  wires:
  Resistance/1 -> R/1

== system H8_6gdl_hil/EMS/RL3/Subsystem ==
  Current : Inport
  Temperature : Inport  Port=2
  Resistance : Constant  Value=ems.Resistance
  R : Outport
  wires:
  Resistance/1 -> R/1

== system H8_6gdl_hil/HEMS1/RL/Subsystem ==
  Current : Inport
  Temperature : Inport  Port=2
  Resistance : Constant  Value=hems.Resistance
  R : Outport
  wires:
  Resistance/1 -> R/1

== system H8_6gdl_hil/HEMS1/RL1/Subsystem ==
  Current : Inport
  Temperature : Inport  Port=2
  Resistance : Constant  Value=hems.Resistance
  R : Outport
  wires:
  Resistance/1 -> R/1

== system H8_6gdl_hil/HEMS1/RL2/Subsystem ==
  Current : Inport
  Temperature : Inport  Port=2
  Resistance : Constant  Value=hems.Resistance
  R : Outport
  wires:
  Resistance/1 -> R/1

== system H8_6gdl_hil/HEMS1/RL3/Subsystem ==
  Current : Inport
  Temperature : Inport  Port=2
  Resistance : Constant  Value=hems.Resistance
  R : Outport
  wires:
  Resistance/1 -> R/1

== system H8_6gdl_hil/Modelado electromagnetico/Guidance/power_ems1 ==
  I : Inport
  Constant8 : Constant  Value=ems.Resistance
  Power : Math  Operator=magnitude^2
  Product : Product
  p(t) : Outport
  wires:
  I/1 -> Power/1
  Product/1 -> p(t)/1
  Power/1 -> Product/1
  Constant8/1 -> Product/2
